simulink model "test_cosimulation"  (Simulink 7.4)
settings: Solver=ode45  StartTime=0.0  StopTime=15.0  FixedStep=0.01  RelTol=1e-3
libraries: instrumentlib x2
settings Model: Creator=tasora  LastModifiedBy=tasora

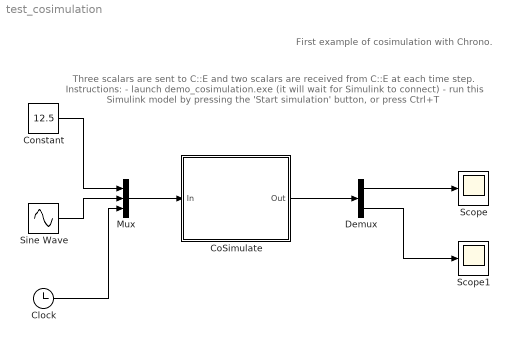
== system test_cosimulation ==
  note: Three scalars are sent to C::E and two scalars are received from C::E
      | at each time step.
      | Instructions:
      | - launch demo_cosimulation.exe (it will wait for Simulink to connect)
      | - run this Simulink model by pressing the 'Start simulation' button, or press Ctrl+T
  note: First example of cosimulation with Chrono.
  Clock : Clock
      settings: Decimation=10
  CoSimulate : Subsystem  Description=|  mask{com_step=0.2, tcp_data_size=2, host_name=localhost, tcp_port=50009, tcp_timeout=15}
      | This block can be used to exchange data with Chrono.                                                                                             
      | A Chrono program with a running ChCosimulation interface must be started, it will work as a server; then the Simulink program must be run.
      | Note! check that the         dimensions of the exchanged vectors do match!
      mask prompts: com_step "Communication step size"; tcp_data_size "N. of scalars received from C::E (as block output)"; host_name "TCP host name (ex. 'localhost', or 'www.myhost.com')"; tcp_port "TCP port (ex. 50007)"; tcp_timeout "TCP timeout (seconds)"
      mask init:
      | block_receive = [gcb, '/TCP Receive'];
      | set_param(block_receive, 'SampleTime', num2str(com_step));
      | set_param(block_receive, 'Host', host_name);
      | set_param(block_receive, 'Port', num2str(tcp_port));
      | set_param(block_receive, 'DataSize', num2str(tcp_data_size+1));
      | set_param(block_receive, 'Timeout', num2str(tcp_timeout));
      | block_send = [gcb, '/TCP Send'];
      | set_param(block_send, 'Host', host_name);
      | set_param(block_send, 'Port', num2str(tcp_port));
      mask Display:
      | image(imread('block_logo.png'))
      | disp('C::E                   ')
  Constant : Constant  Value=12.5  OutDataType=fixdt(1, 16)  OutScaling=2^0
  Demux : Demux  Outputs=2
  Mux : Mux  Inputs=3
  Scope : Scope
  Scope1 : Scope
  Sine Wave : Sin  Amplitude=5  Bias=0  Frequency=0.5  Phase=0  Samples=10  SampleTime=0  Offset=0
  wires:
  Constant/1 -> Mux/1
  Sine Wave/1 -> Mux/2
  Clock/1 -> Mux/3
  Mux/1 -> CoSimulate/1(In)
  CoSimulate/1(Out) -> Demux/1
  Demux/1 -> Scope/1
  Demux/2 -> Scope1/1

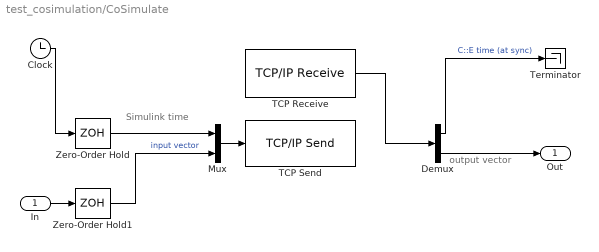
== system test_cosimulation/CoSimulate ==
  note: output vector
  note: Simulink time
  In : Inport
  Clock : Clock
      settings: Decimation=10
  Demux : Demux  Outputs=[1 -1]
  Mux : Mux  Inputs=2
  TCP Receive : instrumentlib/TCP//IP Receive  Priority=1  DialogController=instrumentcreatedialog  DialogControllerArgs=DataTag0  Host=localhost  Port=50009  DataSize=3  EnableBlockingMode=on  Timeout=15  SampleTime=0.2  DataType=double  ByteOrder=LittleEndian
  TCP Send : instrumentlib/TCP//IP Send  Priority=2  DialogController=instrumentcreatedialog  DialogControllerArgs=DataTag1  Host=localhost  Port=50009  EnableBlockingMode=off  Timeout=10  ByteOrder=LittleEndian
  Terminator : Terminator
  Zero-Order Hold : ZeroOrderHold  SampleTime=com_step
  Zero-Order Hold1 : ZeroOrderHold  SampleTime=com_step
  Out : Outport
  wires:
  Zero-Order Hold/1 -> Mux/1
  Zero-Order Hold1/1 -> Mux/2  "input vector"
  Mux/1 -> TCP Send/1
  Clock/1 -> Zero-Order Hold/1
  In/1 -> Zero-Order Hold1/1
  TCP Receive/1 -> Demux/1
  Demux/1 -> Terminator/1  "C::E time (at sync)"
  Demux/2 -> Out/1
